simulink model "compare_serial"  (R2012b)
settings: Solver=FixedStepDiscrete  SolverMode=SingleTasking  StartTime=0.0  StopTime=5000  FixedStep=1  RelTol=1e-3
libraries: xbsIndex_r4 x1495, xps_library x1, casper_library_misc x1
(part 2 of 15)

== system compare_serial/dec_fir ==
  sync_in : Inport
  real1 : Inport  Port=2
  imag1 : Inport  Port=3
  real2 : Inport  Port=4
  imag2 : Inport  Port=5
  real3 : Inport  Port=6
  imag3 : Inport  Port=7
  real4 : Inport  Port=8
  imag4 : Inport  Port=9
  real5 : Inport  Port=10
  imag5 : Inport  Port=11
  real6 : Inport  Port=12
  imag6 : Inport  Port=13
  real7 : Inport  Port=14
  imag7 : Inport  Port=15
  real8 : Inport  Port=16
  imag8 : Inport  Port=17
  convert1 : xbsIndex_r4/Convert  gui_display_data_type=Fixed-point  arith_type="Signed  (2's comp)"  n_bits=34  bin_pt=24  float_type=Single  exp_bits=8  fraction_bits=24  quantization="Round  (unbiased: +/- Inf)"  overflow=Wrap  en=off  latency=2  dbl_ovrd=off  pipeline=off  block_type=convert
  convert2 : xbsIndex_r4/Convert  gui_display_data_type=Fixed-point  arith_type="Signed  (2's comp)"  n_bits=34  bin_pt=24  float_type=Single  exp_bits=8  fraction_bits=24  quantization="Round  (unbiased: +/- Inf)"  overflow=Wrap  en=off  latency=2  dbl_ovrd=off  pipeline=off  block_type=convert
  delay : xbsIndex_r4/Delay  rst=off  infoeditControl=Selection of Reset will increase slice count due to use of real FFs and instead of SRLs  en=off  latency=8  dbl_ovrd=off  reg_retiming=off  block_type=delay
  fir_dbl_col1 : Subsystem  AncestorBlock=casper_library_downconverter/fir_dbl_col  mask(fir_dbl_col){n_inputs=8, coeff=[3.6558e-05  8.0913e-05  0.00010847   0.0001179  0.00011054  8.9835e-05  6.0569e-05  0.00018614], add_latency=1, mult_latency=2, coeff_bit_width=16, coeff_bin_pt=15, first_stage_hdl=off, adder_imp=Behavioral}
      mask prompts: n_inputs "Inputs"; coeff "Coefficients"; add_latency "Add latency"; mult_latency "Mult Latency"; coeff_bit_width "Coefficient bit width"; coeff_bin_pt "Coefficient binary point"; first_stage_hdl "Implement first stage of adder trees on output as behavioural HDL"; adder_imp "Adder implementation"
      mask init:
      | fir_dbl_col_init(gcb, ...
      |     'n_inputs', n_inputs, ...
      |     'coeff', coeff, ...
      |     'mult_latency', mult_latency, ...
      |     'add_latency', add_latency, ...
      |     'coeff_bit_width', coeff_bit_width, ...
      |     'coeff_bin_pt', coeff_bin_pt,  ...
      |     'first_stage_hdl', first_stage_hdl, ...
      |     'adder_imp', adder_imp);
      mask Help: eval('xlWeb(''http://casper.berkeley.edu/wiki/Fir_dbl_col'')')
      mask TypeOptions adder_imp: Behavioral | Fabric | DSP48
  fir_dbl_col10 : Subsystem  AncestorBlock=casper_library_downconverter/fir_dbl_col  mask(fir_dbl_col){n_inputs=8, coeff=[-0.0039158  -0.0027465  -0.0013032  0.00020791    0.001586   0.0026617   0.0033165    0.003495], add_latency=1, mult_latency=2, coeff_bit_width=16, coeff_bin_pt=15, first_stage_hdl=off, adder_imp=Behavioral}
      mask prompts: n_inputs "Inputs"; coeff "Coefficients"; add_latency "Add latency"; mult_latency "Mult Latency"; coeff_bit_width "Coefficient bit width"; coeff_bin_pt "Coefficient binary point"; first_stage_hdl "Implement first stage of adder trees on output as behavioural HDL"; adder_imp "Adder implementation"
      mask init: same as compare_serial/dec_fir/fir_dbl_col1
      mask Help: eval('xlWeb(''http://casper.berkeley.edu/wiki/Fir_dbl_col'')')
      mask TypeOptions adder_imp: Behavioral | Fabric | DSP48
  fir_dbl_col11 : Subsystem  AncestorBlock=casper_library_downconverter/fir_dbl_col  mask(fir_dbl_col){n_inputs=8, coeff=[0.0045348   0.0026836   0.0006186  -0.0013783  -0.0030542  -0.0042152  -0.0047479  -0.0046275], add_latency=1, mult_latency=2, coeff_bit_width=16, coeff_bin_pt=15, first_stage_hdl=off, adder_imp=Behavioral}
      mask prompts: n_inputs "Inputs"; coeff "Coefficients"; add_latency "Add latency"; mult_latency "Mult Latency"; coeff_bit_width "Coefficient bit width"; coeff_bin_pt "Coefficient binary point"; first_stage_hdl "Implement first stage of adder trees on output as behavioural HDL"; adder_imp "Adder implementation"
      mask init: same as compare_serial/dec_fir/fir_dbl_col1
      mask Help: eval('xlWeb(''http://casper.berkeley.edu/wiki/Fir_dbl_col'')')
      mask TypeOptions adder_imp: Behavioral | Fabric | DSP48
  fir_dbl_col12 : Subsystem  AncestorBlock=casper_library_downconverter/fir_dbl_col  mask(fir_dbl_col){n_inputs=8, coeff=[-0.0049463  -0.0021372  0.00072915   0.0032813   0.0052161   0.0063317   0.0065461   0.0058982], add_latency=1, mult_latency=2, coeff_bit_width=16, coeff_bin_pt=15, first_stage_hdl=off, adder_imp=Behavioral}
      mask prompts: n_inputs "Inputs"; coeff "Coefficients"; add_latency "Add latency"; mult_latency "Mult Latency"; coeff_bit_width "Coefficient bit width"; coeff_bin_pt "Coefficient binary point"; first_stage_hdl "Implement first stage of adder trees on output as behavioural HDL"; adder_imp "Adder implementation"
      mask init: same as compare_serial/dec_fir/fir_dbl_col1
      mask Help: eval('xlWeb(''http://casper.berkeley.edu/wiki/Fir_dbl_col'')')
      mask TypeOptions adder_imp: Behavioral | Fabric | DSP48
  fir_dbl_col13 : Subsystem  AncestorBlock=casper_library_downconverter/fir_dbl_col  mask(fir_dbl_col){n_inputs=8, coeff=[0.0049631  0.00074424  -0.0031897  -0.0063683  -0.0084557  -0.0092805  -0.0088434  -0.0073036], add_latency=1, mult_latency=2, coeff_bit_width=16, coeff_bin_pt=15, first_stage_hdl=off, adder_imp=Behavioral}
      mask prompts: n_inputs "Inputs"; coeff "Coefficients"; add_latency "Add latency"; mult_latency "Mult Latency"; coeff_bit_width "Coefficient bit width"; coeff_bin_pt "Coefficient binary point"; first_stage_hdl "Implement first stage of adder trees on output as behavioural HDL"; adder_imp "Adder implementation"
      mask init: same as compare_serial/dec_fir/fir_dbl_col1
      mask Help: eval('xlWeb(''http://casper.berkeley.edu/wiki/Fir_dbl_col'')')
      mask TypeOptions adder_imp: Behavioral | Fabric | DSP48
  fir_dbl_col14 : Subsystem  AncestorBlock=casper_library_downconverter/fir_dbl_col  mask(fir_dbl_col){n_inputs=8, coeff=[-0.0041692   0.0024096   0.0079096    0.011788    0.013751    0.013761    0.012018   0.0089121], add_latency=1, mult_latency=2, coeff_bit_width=16, coeff_bin_pt=15, first_stage_hdl=off, adder_imp=Behavioral}
      mask prompts: n_inputs "Inputs"; coeff "Coefficients"; add_latency "Add latency"; mult_latency "Mult Latency"; coeff_bit_width "Coefficient bit width"; coeff_bin_pt "Coefficient binary point"; first_stage_hdl "Implement first stage of adder trees on output as behavioural HDL"; adder_imp "Adder implementation"
      mask init: same as compare_serial/dec_fir/fir_dbl_col1
      mask Help: eval('xlWeb(''http://casper.berkeley.edu/wiki/Fir_dbl_col'')')
      mask TypeOptions adder_imp: Behavioral | Fabric | DSP48
  fir_dbl_col15 : Subsystem  AncestorBlock=casper_library_downconverter/fir_dbl_col  mask(fir_dbl_col){n_inputs=8, coeff=[0.00081481   -0.011166   -0.019458   -0.023888   -0.024646   -0.022238   -0.017414   -0.011075], add_latency=1, mult_latency=2, coeff_bit_width=16, coeff_bin_pt=15, first_stage_hdl=off, adder_imp=Behavioral}
      mask prompts: n_inputs "Inputs"; coeff "Coefficients"; add_latency "Add latency"; mult_latency "Mult Latency"; coeff_bit_width "Coefficient bit width"; coeff_bin_pt "Coefficient binary point"; first_stage_hdl "Implement first stage of adder trees on output as behavioural HDL"; adder_imp "Adder implementation"
      mask init: same as compare_serial/dec_fir/fir_dbl_col1
      mask Help: eval('xlWeb(''http://casper.berkeley.edu/wiki/Fir_dbl_col'')')
      mask TypeOptions adder_imp: Behavioral | Fabric | DSP48
  fir_dbl_col16 : Subsystem  AncestorBlock=casper_library_downconverter/fir_dbl_col  mask(fir_dbl_col){n_inputs=8, coeff=[0.11608     0.11089     0.10094    0.087016    0.070234    0.051888    0.033353    0.015947], add_latency=1, mult_latency=2, coeff_bit_width=16, coeff_bin_pt=15, first_stage_hdl=off, adder_imp=Behavioral}
      mask prompts: n_inputs "Inputs"; coeff "Coefficients"; add_latency "Add latency"; mult_latency "Mult Latency"; coeff_bit_width "Coefficient bit width"; coeff_bin_pt "Coefficient binary point"; first_stage_hdl "Implement first stage of adder trees on output as behavioural HDL"; adder_imp "Adder implementation"
      mask init: same as compare_serial/dec_fir/fir_dbl_col1
      mask Help: eval('xlWeb(''http://casper.berkeley.edu/wiki/Fir_dbl_col'')')
      mask TypeOptions adder_imp: Behavioral | Fabric | DSP48
  fir_dbl_col2 : Subsystem  AncestorBlock=casper_library_downconverter/fir_dbl_col  mask(fir_dbl_col){n_inputs=8, coeff=[-0.0001139 -0.00017961 -0.00021408 -0.00021652 -0.00019053 -0.00014309 -8.3201e-05 -2.0412e-05], add_latency=1, mult_latency=2, coeff_bit_width=16, coeff_bin_pt=15, first_stage_hdl=off, adder_imp=Behavioral}
      mask prompts: n_inputs "Inputs"; coeff "Coefficients"; add_latency "Add latency"; mult_latency "Mult Latency"; coeff_bit_width "Coefficient bit width"; coeff_bin_pt "Coefficient binary point"; first_stage_hdl "Implement first stage of adder trees on output as behavioural HDL"; adder_imp "Adder implementation"
      mask init: same as compare_serial/dec_fir/fir_dbl_col1
      mask Help: eval('xlWeb(''http://casper.berkeley.edu/wiki/Fir_dbl_col'')')
      mask TypeOptions adder_imp: Behavioral | Fabric | DSP48
  fir_dbl_col3 : Subsystem  AncestorBlock=casper_library_downconverter/fir_dbl_col  mask(fir_dbl_col){n_inputs=8, coeff=[0.0002565  0.00034013  0.00037076  0.00035001  0.00028615  0.00019229  8.4099e-05 -2.2589e-05], add_latency=1, mult_latency=2, coeff_bit_width=16, coeff_bin_pt=15, first_stage_hdl=off, adder_imp=Behavioral}
      mask prompts: n_inputs "Inputs"; coeff "Coefficients"; add_latency "Add latency"; mult_latency "Mult Latency"; coeff_bit_width "Coefficient bit width"; coeff_bin_pt "Coefficient binary point"; first_stage_hdl "Implement first stage of adder trees on output as behavioural HDL"; adder_imp "Adder implementation"
      mask init: same as compare_serial/dec_fir/fir_dbl_col1
      mask Help: eval('xlWeb(''http://casper.berkeley.edu/wiki/Fir_dbl_col'')')
      mask TypeOptions adder_imp: Behavioral | Fabric | DSP48
  fir_dbl_col4 : Subsystem  AncestorBlock=casper_library_downconverter/fir_dbl_col  mask(fir_dbl_col){n_inputs=8, coeff=[-0.00048623 -0.00057488 -0.00058051 -0.00051035 -0.00038093 -0.00021502  -3.797e-05  0.00012591], add_latency=1, mult_latency=2, coeff_bit_width=16, coeff_bin_pt=15, first_stage_hdl=off, adder_imp=Behavioral}
      mask prompts: n_inputs "Inputs"; coeff "Coefficients"; add_latency "Add latency"; mult_latency "Mult Latency"; coeff_bit_width "Coefficient bit width"; coeff_bin_pt "Coefficient binary point"; first_stage_hdl "Implement first stage of adder trees on output as behavioural HDL"; adder_imp "Adder implementation"
      mask init: same as compare_serial/dec_fir/fir_dbl_col1
      mask Help: eval('xlWeb(''http://casper.berkeley.edu/wiki/Fir_dbl_col'')')
      mask TypeOptions adder_imp: Behavioral | Fabric | DSP48
  fir_dbl_col5 : Subsystem  AncestorBlock=casper_library_downconverter/fir_dbl_col  mask(fir_dbl_col){n_inputs=8, coeff=[0.00082138  0.00088865  0.00083479  0.00067746   0.0004464  0.00017839 -8.8198e-05 -0.00031866], add_latency=1, mult_latency=2, coeff_bit_width=16, coeff_bin_pt=15, first_stage_hdl=off, adder_imp=Behavioral}
      mask prompts: n_inputs "Inputs"; coeff "Coefficients"; add_latency "Add latency"; mult_latency "Mult Latency"; coeff_bit_width "Coefficient bit width"; coeff_bin_pt "Coefficient binary point"; first_stage_hdl "Implement first stage of adder trees on output as behavioural HDL"; adder_imp "Adder implementation"
      mask init: same as compare_serial/dec_fir/fir_dbl_col1
      mask Help: eval('xlWeb(''http://casper.berkeley.edu/wiki/Fir_dbl_col'')')
      mask TypeOptions adder_imp: Behavioral | Fabric | DSP48
  fir_dbl_col6 : Subsystem  AncestorBlock=casper_library_downconverter/fir_dbl_col  mask(fir_dbl_col){n_inputs=8, coeff=[-0.0012722  -0.0012742  -0.0011107 -0.00081658  -0.0004409 -3.9415e-05  0.00033331  0.00063107], add_latency=1, mult_latency=2, coeff_bit_width=16, coeff_bin_pt=15, first_stage_hdl=off, adder_imp=Behavioral}
      mask prompts: n_inputs "Inputs"; coeff "Coefficients"; add_latency "Add latency"; mult_latency "Mult Latency"; coeff_bit_width "Coefficient bit width"; coeff_bin_pt "Coefficient binary point"; first_stage_hdl "Implement first stage of adder trees on output as behavioural HDL"; adder_imp "Adder implementation"
      mask init: same as compare_serial/dec_fir/fir_dbl_col1
      mask Help: eval('xlWeb(''http://casper.berkeley.edu/wiki/Fir_dbl_col'')')
      mask TypeOptions adder_imp: Behavioral | Fabric | DSP48
  fir_dbl_col7 : Subsystem  AncestorBlock=casper_library_downconverter/fir_dbl_col  mask(fir_dbl_col){n_inputs=8, coeff=[0.0018361   0.0017079   0.0013679  0.00087646  0.00030942 -0.00025349  -0.0007392  -0.0010905], add_latency=1, mult_latency=2, coeff_bit_width=16, coeff_bin_pt=15, first_stage_hdl=off, adder_imp=Behavioral}
      mask prompts: n_inputs "Inputs"; coeff "Coefficients"; add_latency "Add latency"; mult_latency "Mult Latency"; coeff_bit_width "Coefficient bit width"; coeff_bin_pt "Coefficient binary point"; first_stage_hdl "Implement first stage of adder trees on output as behavioural HDL"; adder_imp "Adder implementation"
      mask init: same as compare_serial/dec_fir/fir_dbl_col1
      mask Help: eval('xlWeb(''http://casper.berkeley.edu/wiki/Fir_dbl_col'')')
      mask TypeOptions adder_imp: Behavioral | Fabric | DSP48
  fir_dbl_col8 : Subsystem  AncestorBlock=casper_library_downconverter/fir_dbl_col  mask(fir_dbl_col){n_inputs=8, coeff=[-0.0024941  -0.0021466  -0.0015457 -0.00078824   1.582e-05  0.00075832   0.0013471    0.001717], add_latency=1, mult_latency=2, coeff_bit_width=16, coeff_bin_pt=15, first_stage_hdl=off, adder_imp=Behavioral}
      mask prompts: n_inputs "Inputs"; coeff "Coefficients"; add_latency "Add latency"; mult_latency "Mult Latency"; coeff_bit_width "Coefficient bit width"; coeff_bin_pt "Coefficient binary point"; first_stage_hdl "Implement first stage of adder trees on output as behavioural HDL"; adder_imp "Adder implementation"
      mask init: same as compare_serial/dec_fir/fir_dbl_col1
      mask Help: eval('xlWeb(''http://casper.berkeley.edu/wiki/Fir_dbl_col'')')
      mask TypeOptions adder_imp: Behavioral | Fabric | DSP48
  fir_dbl_col9 : Subsystem  AncestorBlock=casper_library_downconverter/fir_dbl_col  mask(fir_dbl_col){n_inputs=8, coeff=[0.0032074   0.0025239   0.0015612  0.00046403 -0.00061536  -0.0015379  -0.0021949  -0.0025197], add_latency=1, mult_latency=2, coeff_bit_width=16, coeff_bin_pt=15, first_stage_hdl=off, adder_imp=Behavioral}
      mask prompts: n_inputs "Inputs"; coeff "Coefficients"; add_latency "Add latency"; mult_latency "Mult Latency"; coeff_bit_width "Coefficient bit width"; coeff_bin_pt "Coefficient binary point"; first_stage_hdl "Implement first stage of adder trees on output as behavioural HDL"; adder_imp "Adder implementation"
      mask init: same as compare_serial/dec_fir/fir_dbl_col1
      mask Help: eval('xlWeb(''http://casper.berkeley.edu/wiki/Fir_dbl_col'')')
      mask TypeOptions adder_imp: Behavioral | Fabric | DSP48
  imag_sum : Subsystem  AncestorBlock=casper_library_misc/adder_tree  mask(adder_tree){n_inputs=16, latency=1, adder_imp=Behavioral, first_stage_hdl=off}
      mask prompts: n_inputs "Number of Inputs"; latency "Add Latency"; adder_imp "Adder implementation"; first_stage_hdl "Use behavioural HDL for first stage of adders"
      mask help:
      | Sums all inputs using a tree of adds and delays.
      |
      | Number of inputs: The number of inputs to the block to be summed
      | Add latency: The number of clock cycles to perform one addition (affects timing)..
      | Adder implementation: choice of fabric or DSP48E core, or behavioral HDL
      | Use behavioural HDL for first stage of adders: Causes the first stage of adders to be absorbed into DSP blocks if multipliers precede them (Virtex 5). Overrides Adder implementation
      mask init:
      | adder_tree_init(gcb, ...
      |     'n_inputs', n_inputs, ...
      |     'latency', latency, ...
      |     'adder_imp', adder_imp, ...
      |     'first_stage_hdl', first_stage_hdl);
      settings: AttributesFormatString=latency 4
      mask Help: eval('xlWeb(''http://casper.berkeley.edu/wiki/Adder_tree'')')
      mask TypeOptions adder_imp: Behavioral | Fabric | DSP48
  real_sum : Subsystem  AncestorBlock=casper_library_misc/adder_tree  mask(adder_tree){n_inputs=16, latency=1, adder_imp=Behavioral, first_stage_hdl=off}
      mask prompts: n_inputs "Number of Inputs"; latency "Add Latency"; adder_imp "Adder implementation"; first_stage_hdl "Use behavioural HDL for first stage of adders"
      mask help:
      | Sums all inputs using a tree of adds and delays.
      |
      | Number of inputs: The number of inputs to the block to be summed
      | Add latency: The number of clock cycles to perform one addition (affects timing)..
      | Adder implementation: choice of fabric or DSP48E core, or behavioral HDL
      | Use behavioural HDL for first stage of adders: Causes the first stage of adders to be absorbed into DSP blocks if multipliers precede them (Virtex 5). Overrides Adder implementation
      mask init:
      | adder_tree_init(gcb, ...
      |     'n_inputs', n_inputs, ...
      |     'latency', latency, ...
      |     'adder_imp', adder_imp, ...
      |     'first_stage_hdl', first_stage_hdl);
      settings: AttributesFormatString=latency 4
      mask Help: eval('xlWeb(''http://casper.berkeley.edu/wiki/Adder_tree'')')
      mask TypeOptions adder_imp: Behavioral | Fabric | DSP48
  ri_to_c : casper_library_misc/ri_to_c
  shift1 : xbsIndex_r4/Shift  shift_dir=Left  shift_bits=0  en=off  latency=0  precision=Full  arith_type="Signed  (2's comp)"  n_bits=16  bin_pt=14  quantization=Truncate  overflow=Wrap  dbl_ovrd=off  block_type=shift
  shift2 : xbsIndex_r4/Shift  shift_dir=Left  shift_bits=0  en=off  latency=0  precision=Full  arith_type="Signed  (2's comp)"  n_bits=16  bin_pt=14  quantization=Truncate  overflow=Wrap  dbl_ovrd=off  block_type=shift
  sync_out : Outport
  dout : Outport  Port=2
  wires:
  real1/1 -> fir_dbl_col1/1(real1)
  imag1/1 -> fir_dbl_col1/2(imag1)
  real2/1 -> fir_dbl_col1/3(real2)
  imag2/1 -> fir_dbl_col1/4(imag2)
  real3/1 -> fir_dbl_col1/5(real3)
  imag3/1 -> fir_dbl_col1/6(imag3)
  real4/1 -> fir_dbl_col1/7(real4)
  imag4/1 -> fir_dbl_col1/8(imag4)
  real5/1 -> fir_dbl_col1/9(real5)
  imag5/1 -> fir_dbl_col1/10(imag5)
  real6/1 -> fir_dbl_col1/11(real6)
  imag6/1 -> fir_dbl_col1/12(imag6)
  real7/1 -> fir_dbl_col1/13(real7)
  imag7/1 -> fir_dbl_col1/14(imag7)
  real8/1 -> fir_dbl_col1/15(real8)
  imag8/1 -> fir_dbl_col1/16(imag8)
  fir_dbl_col1/33(real_sum) -> real_sum/2(din1)
  fir_dbl_col1/34(imag_sum) -> imag_sum/2(din1)
  fir_dbl_col1/1(real_out1) -> fir_dbl_col2/1(real1)
  fir_dbl_col1/2(imag_out1) -> fir_dbl_col2/2(imag1)
  fir_dbl_col1/3(real_out2) -> fir_dbl_col2/3(real2)
  fir_dbl_col1/4(imag_out2) -> fir_dbl_col2/4(imag2)
  fir_dbl_col1/5(real_out3) -> fir_dbl_col2/5(real3)
  fir_dbl_col1/6(imag_out3) -> fir_dbl_col2/6(imag3)
  fir_dbl_col1/7(real_out4) -> fir_dbl_col2/7(real4)
  fir_dbl_col1/8(imag_out4) -> fir_dbl_col2/8(imag4)
  fir_dbl_col1/9(real_out5) -> fir_dbl_col2/9(real5)
  fir_dbl_col1/10(imag_out5) -> fir_dbl_col2/10(imag5)
  fir_dbl_col1/11(real_out6) -> fir_dbl_col2/11(real6)
  fir_dbl_col1/12(imag_out6) -> fir_dbl_col2/12(imag6)
  fir_dbl_col1/13(real_out7) -> fir_dbl_col2/13(real7)
  fir_dbl_col1/14(imag_out7) -> fir_dbl_col2/14(imag7)
  fir_dbl_col1/15(real_out8) -> fir_dbl_col2/15(real8)
  fir_dbl_col1/16(imag_out8) -> fir_dbl_col2/16(imag8)
  fir_dbl_col2/33(real_sum) -> real_sum/3(din2)
  fir_dbl_col2/34(imag_sum) -> imag_sum/3(din2)
  fir_dbl_col2/1(real_out1) -> fir_dbl_col3/1(real1)
  fir_dbl_col2/2(imag_out1) -> fir_dbl_col3/2(imag1)
  fir_dbl_col2/3(real_out2) -> fir_dbl_col3/3(real2)
  fir_dbl_col2/4(imag_out2) -> fir_dbl_col3/4(imag2)
  fir_dbl_col2/5(real_out3) -> fir_dbl_col3/5(real3)
  fir_dbl_col2/6(imag_out3) -> fir_dbl_col3/6(imag3)
  fir_dbl_col2/7(real_out4) -> fir_dbl_col3/7(real4)
  fir_dbl_col2/8(imag_out4) -> fir_dbl_col3/8(imag4)
  fir_dbl_col2/9(real_out5) -> fir_dbl_col3/9(real5)
  fir_dbl_col2/10(imag_out5) -> fir_dbl_col3/10(imag5)
  fir_dbl_col2/11(real_out6) -> fir_dbl_col3/11(real6)
  fir_dbl_col2/12(imag_out6) -> fir_dbl_col3/12(imag6)
  fir_dbl_col2/13(real_out7) -> fir_dbl_col3/13(real7)
  fir_dbl_col2/14(imag_out7) -> fir_dbl_col3/14(imag7)
  fir_dbl_col2/15(real_out8) -> fir_dbl_col3/15(real8)
  fir_dbl_col2/16(imag_out8) -> fir_dbl_col3/16(imag8)
  fir_dbl_col3/33(real_sum) -> real_sum/4(din3)
  fir_dbl_col3/34(imag_sum) -> imag_sum/4(din3)
  fir_dbl_col3/1(real_out1) -> fir_dbl_col4/1(real1)
  fir_dbl_col3/2(imag_out1) -> fir_dbl_col4/2(imag1)
  fir_dbl_col3/3(real_out2) -> fir_dbl_col4/3(real2)
  fir_dbl_col3/4(imag_out2) -> fir_dbl_col4/4(imag2)
  fir_dbl_col3/5(real_out3) -> fir_dbl_col4/5(real3)
  fir_dbl_col3/6(imag_out3) -> fir_dbl_col4/6(imag3)
  fir_dbl_col3/7(real_out4) -> fir_dbl_col4/7(real4)
  fir_dbl_col3/8(imag_out4) -> fir_dbl_col4/8(imag4)
  fir_dbl_col3/9(real_out5) -> fir_dbl_col4/9(real5)
  fir_dbl_col3/10(imag_out5) -> fir_dbl_col4/10(imag5)
  fir_dbl_col3/11(real_out6) -> fir_dbl_col4/11(real6)
  fir_dbl_col3/12(imag_out6) -> fir_dbl_col4/12(imag6)
  fir_dbl_col3/13(real_out7) -> fir_dbl_col4/13(real7)
  fir_dbl_col3/14(imag_out7) -> fir_dbl_col4/14(imag7)
  fir_dbl_col3/15(real_out8) -> fir_dbl_col4/15(real8)
  fir_dbl_col3/16(imag_out8) -> fir_dbl_col4/16(imag8)
  fir_dbl_col4/33(real_sum) -> real_sum/5(din4)
  fir_dbl_col4/34(imag_sum) -> imag_sum/5(din4)
  fir_dbl_col4/1(real_out1) -> fir_dbl_col5/1(real1)
  fir_dbl_col4/2(imag_out1) -> fir_dbl_col5/2(imag1)
  fir_dbl_col4/3(real_out2) -> fir_dbl_col5/3(real2)
  fir_dbl_col4/4(imag_out2) -> fir_dbl_col5/4(imag2)
  fir_dbl_col4/5(real_out3) -> fir_dbl_col5/5(real3)
  fir_dbl_col4/6(imag_out3) -> fir_dbl_col5/6(imag3)
  fir_dbl_col4/7(real_out4) -> fir_dbl_col5/7(real4)
  fir_dbl_col4/8(imag_out4) -> fir_dbl_col5/8(imag4)
  fir_dbl_col4/9(real_out5) -> fir_dbl_col5/9(real5)
  fir_dbl_col4/10(imag_out5) -> fir_dbl_col5/10(imag5)
  fir_dbl_col4/11(real_out6) -> fir_dbl_col5/11(real6)
  fir_dbl_col4/12(imag_out6) -> fir_dbl_col5/12(imag6)
  fir_dbl_col4/13(real_out7) -> fir_dbl_col5/13(real7)
  fir_dbl_col4/14(imag_out7) -> fir_dbl_col5/14(imag7)
  fir_dbl_col4/15(real_out8) -> fir_dbl_col5/15(real8)
  fir_dbl_col4/16(imag_out8) -> fir_dbl_col5/16(imag8)
  fir_dbl_col5/33(real_sum) -> real_sum/6(din5)
  fir_dbl_col5/34(imag_sum) -> imag_sum/6(din5)
  fir_dbl_col5/1(real_out1) -> fir_dbl_col6/1(real1)
  fir_dbl_col5/2(imag_out1) -> fir_dbl_col6/2(imag1)
  fir_dbl_col5/3(real_out2) -> fir_dbl_col6/3(real2)
  fir_dbl_col5/4(imag_out2) -> fir_dbl_col6/4(imag2)
  fir_dbl_col5/5(real_out3) -> fir_dbl_col6/5(real3)
  fir_dbl_col5/6(imag_out3) -> fir_dbl_col6/6(imag3)
  fir_dbl_col5/7(real_out4) -> fir_dbl_col6/7(real4)
  fir_dbl_col5/8(imag_out4) -> fir_dbl_col6/8(imag4)
  fir_dbl_col5/9(real_out5) -> fir_dbl_col6/9(real5)
  fir_dbl_col5/10(imag_out5) -> fir_dbl_col6/10(imag5)
  fir_dbl_col5/11(real_out6) -> fir_dbl_col6/11(real6)
  fir_dbl_col5/12(imag_out6) -> fir_dbl_col6/12(imag6)
  fir_dbl_col5/13(real_out7) -> fir_dbl_col6/13(real7)
  fir_dbl_col5/14(imag_out7) -> fir_dbl_col6/14(imag7)
  fir_dbl_col5/15(real_out8) -> fir_dbl_col6/15(real8)
  fir_dbl_col5/16(imag_out8) -> fir_dbl_col6/16(imag8)
  fir_dbl_col6/33(real_sum) -> real_sum/7(din6)
  fir_dbl_col6/34(imag_sum) -> imag_sum/7(din6)
  fir_dbl_col6/1(real_out1) -> fir_dbl_col7/1(real1)
  fir_dbl_col6/2(imag_out1) -> fir_dbl_col7/2(imag1)
  fir_dbl_col6/3(real_out2) -> fir_dbl_col7/3(real2)
  fir_dbl_col6/4(imag_out2) -> fir_dbl_col7/4(imag2)
  fir_dbl_col6/5(real_out3) -> fir_dbl_col7/5(real3)
  fir_dbl_col6/6(imag_out3) -> fir_dbl_col7/6(imag3)
  fir_dbl_col6/7(real_out4) -> fir_dbl_col7/7(real4)
  fir_dbl_col6/8(imag_out4) -> fir_dbl_col7/8(imag4)
  fir_dbl_col6/9(real_out5) -> fir_dbl_col7/9(real5)
  fir_dbl_col6/10(imag_out5) -> fir_dbl_col7/10(imag5)
  fir_dbl_col6/11(real_out6) -> fir_dbl_col7/11(real6)
  fir_dbl_col6/12(imag_out6) -> fir_dbl_col7/12(imag6)
  fir_dbl_col6/13(real_out7) -> fir_dbl_col7/13(real7)
  fir_dbl_col6/14(imag_out7) -> fir_dbl_col7/14(imag7)
  fir_dbl_col6/15(real_out8) -> fir_dbl_col7/15(real8)
  fir_dbl_col6/16(imag_out8) -> fir_dbl_col7/16(imag8)
  fir_dbl_col7/33(real_sum) -> real_sum/8(din7)
  fir_dbl_col7/34(imag_sum) -> imag_sum/8(din7)
  fir_dbl_col7/1(real_out1) -> fir_dbl_col8/1(real1)
  fir_dbl_col7/2(imag_out1) -> fir_dbl_col8/2(imag1)
  fir_dbl_col7/3(real_out2) -> fir_dbl_col8/3(real2)
  fir_dbl_col7/4(imag_out2) -> fir_dbl_col8/4(imag2)
  fir_dbl_col7/5(real_out3) -> fir_dbl_col8/5(real3)
  fir_dbl_col7/6(imag_out3) -> fir_dbl_col8/6(imag3)
  fir_dbl_col7/7(real_out4) -> fir_dbl_col8/7(real4)
  fir_dbl_col7/8(imag_out4) -> fir_dbl_col8/8(imag4)
  fir_dbl_col7/9(real_out5) -> fir_dbl_col8/9(real5)
  fir_dbl_col7/10(imag_out5) -> fir_dbl_col8/10(imag5)
  fir_dbl_col7/11(real_out6) -> fir_dbl_col8/11(real6)
  fir_dbl_col7/12(imag_out6) -> fir_dbl_col8/12(imag6)
  fir_dbl_col7/13(real_out7) -> fir_dbl_col8/13(real7)
  fir_dbl_col7/14(imag_out7) -> fir_dbl_col8/14(imag7)
  fir_dbl_col7/15(real_out8) -> fir_dbl_col8/15(real8)
  fir_dbl_col7/16(imag_out8) -> fir_dbl_col8/16(imag8)
  fir_dbl_col8/33(real_sum) -> real_sum/9(din8)
  fir_dbl_col8/34(imag_sum) -> imag_sum/9(din8)
  fir_dbl_col8/1(real_out1) -> fir_dbl_col9/1(real1)
  fir_dbl_col8/2(imag_out1) -> fir_dbl_col9/2(imag1)
  fir_dbl_col8/3(real_out2) -> fir_dbl_col9/3(real2)
  fir_dbl_col8/4(imag_out2) -> fir_dbl_col9/4(imag2)
  fir_dbl_col8/5(real_out3) -> fir_dbl_col9/5(real3)
  fir_dbl_col8/6(imag_out3) -> fir_dbl_col9/6(imag3)
  fir_dbl_col8/7(real_out4) -> fir_dbl_col9/7(real4)
  fir_dbl_col8/8(imag_out4) -> fir_dbl_col9/8(imag4)
  fir_dbl_col8/9(real_out5) -> fir_dbl_col9/9(real5)
  fir_dbl_col8/10(imag_out5) -> fir_dbl_col9/10(imag5)
  fir_dbl_col8/11(real_out6) -> fir_dbl_col9/11(real6)
  fir_dbl_col8/12(imag_out6) -> fir_dbl_col9/12(imag6)
  fir_dbl_col8/13(real_out7) -> fir_dbl_col9/13(real7)
  fir_dbl_col8/14(imag_out7) -> fir_dbl_col9/14(imag7)
  fir_dbl_col8/15(real_out8) -> fir_dbl_col9/15(real8)
  fir_dbl_col8/16(imag_out8) -> fir_dbl_col9/16(imag8)
  fir_dbl_col9/33(real_sum) -> real_sum/10(din9)
  fir_dbl_col9/34(imag_sum) -> imag_sum/10(din9)
  fir_dbl_col9/1(real_out1) -> fir_dbl_col10/1(real1)
  fir_dbl_col9/2(imag_out1) -> fir_dbl_col10/2(imag1)
  fir_dbl_col9/3(real_out2) -> fir_dbl_col10/3(real2)
  fir_dbl_col9/4(imag_out2) -> fir_dbl_col10/4(imag2)
  fir_dbl_col9/5(real_out3) -> fir_dbl_col10/5(real3)
  fir_dbl_col9/6(imag_out3) -> fir_dbl_col10/6(imag3)
  fir_dbl_col9/7(real_out4) -> fir_dbl_col10/7(real4)
  fir_dbl_col9/8(imag_out4) -> fir_dbl_col10/8(imag4)
  fir_dbl_col9/9(real_out5) -> fir_dbl_col10/9(real5)
  fir_dbl_col9/10(imag_out5) -> fir_dbl_col10/10(imag5)
  fir_dbl_col9/11(real_out6) -> fir_dbl_col10/11(real6)
  fir_dbl_col9/12(imag_out6) -> fir_dbl_col10/12(imag6)
  fir_dbl_col9/13(real_out7) -> fir_dbl_col10/13(real7)
  fir_dbl_col9/14(imag_out7) -> fir_dbl_col10/14(imag7)
  fir_dbl_col9/15(real_out8) -> fir_dbl_col10/15(real8)
  fir_dbl_col9/16(imag_out8) -> fir_dbl_col10/16(imag8)
  fir_dbl_col10/33(real_sum) -> real_sum/11(din10)
  fir_dbl_col10/34(imag_sum) -> imag_sum/11(din10)
  fir_dbl_col10/1(real_out1) -> fir_dbl_col11/1(real1)
  fir_dbl_col10/2(imag_out1) -> fir_dbl_col11/2(imag1)
  fir_dbl_col10/3(real_out2) -> fir_dbl_col11/3(real2)
  fir_dbl_col10/4(imag_out2) -> fir_dbl_col11/4(imag2)
  fir_dbl_col10/5(real_out3) -> fir_dbl_col11/5(real3)
  fir_dbl_col10/6(imag_out3) -> fir_dbl_col11/6(imag3)
  fir_dbl_col10/7(real_out4) -> fir_dbl_col11/7(real4)
  fir_dbl_col10/8(imag_out4) -> fir_dbl_col11/8(imag4)
  fir_dbl_col10/9(real_out5) -> fir_dbl_col11/9(real5)
  fir_dbl_col10/10(imag_out5) -> fir_dbl_col11/10(imag5)
  fir_dbl_col10/11(real_out6) -> fir_dbl_col11/11(real6)
  fir_dbl_col10/12(imag_out6) -> fir_dbl_col11/12(imag6)
  fir_dbl_col10/13(real_out7) -> fir_dbl_col11/13(real7)
  fir_dbl_col10/14(imag_out7) -> fir_dbl_col11/14(imag7)
  fir_dbl_col10/15(real_out8) -> fir_dbl_col11/15(real8)
  fir_dbl_col10/16(imag_out8) -> fir_dbl_col11/16(imag8)
  fir_dbl_col11/33(real_sum) -> real_sum/12(din11)
  fir_dbl_col11/34(imag_sum) -> imag_sum/12(din11)
  fir_dbl_col11/1(real_out1) -> fir_dbl_col12/1(real1)
  fir_dbl_col11/2(imag_out1) -> fir_dbl_col12/2(imag1)
  fir_dbl_col11/3(real_out2) -> fir_dbl_col12/3(real2)
  fir_dbl_col11/4(imag_out2) -> fir_dbl_col12/4(imag2)
  fir_dbl_col11/5(real_out3) -> fir_dbl_col12/5(real3)
  fir_dbl_col11/6(imag_out3) -> fir_dbl_col12/6(imag3)
  fir_dbl_col11/7(real_out4) -> fir_dbl_col12/7(real4)
  fir_dbl_col11/8(imag_out4) -> fir_dbl_col12/8(imag4)
  fir_dbl_col11/9(real_out5) -> fir_dbl_col12/9(real5)
  fir_dbl_col11/10(imag_out5) -> fir_dbl_col12/10(imag5)
  fir_dbl_col11/11(real_out6) -> fir_dbl_col12/11(real6)
  fir_dbl_col11/12(imag_out6) -> fir_dbl_col12/12(imag6)
  fir_dbl_col11/13(real_out7) -> fir_dbl_col12/13(real7)
  fir_dbl_col11/14(imag_out7) -> fir_dbl_col12/14(imag7)
  fir_dbl_col11/15(real_out8) -> fir_dbl_col12/15(real8)
  fir_dbl_col11/16(imag_out8) -> fir_dbl_col12/16(imag8)
  fir_dbl_col12/33(real_sum) -> real_sum/13(din12)
  fir_dbl_col12/34(imag_sum) -> imag_sum/13(din12)
  fir_dbl_col12/1(real_out1) -> fir_dbl_col13/1(real1)
  fir_dbl_col12/2(imag_out1) -> fir_dbl_col13/2(imag1)
  fir_dbl_col12/3(real_out2) -> fir_dbl_col13/3(real2)
  fir_dbl_col12/4(imag_out2) -> fir_dbl_col13/4(imag2)
  fir_dbl_col12/5(real_out3) -> fir_dbl_col13/5(real3)
  fir_dbl_col12/6(imag_out3) -> fir_dbl_col13/6(imag3)
  fir_dbl_col12/7(real_out4) -> fir_dbl_col13/7(real4)
  fir_dbl_col12/8(imag_out4) -> fir_dbl_col13/8(imag4)
  fir_dbl_col12/9(real_out5) -> fir_dbl_col13/9(real5)
  fir_dbl_col12/10(imag_out5) -> fir_dbl_col13/10(imag5)
  fir_dbl_col12/11(real_out6) -> fir_dbl_col13/11(real6)
  fir_dbl_col12/12(imag_out6) -> fir_dbl_col13/12(imag6)
  fir_dbl_col12/13(real_out7) -> fir_dbl_col13/13(real7)
  fir_dbl_col12/14(imag_out7) -> fir_dbl_col13/14(imag7)
  fir_dbl_col12/15(real_out8) -> fir_dbl_col13/15(real8)
  fir_dbl_col12/16(imag_out8) -> fir_dbl_col13/16(imag8)
  fir_dbl_col13/33(real_sum) -> real_sum/14(din13)
  fir_dbl_col13/34(imag_sum) -> imag_sum/14(din13)
  fir_dbl_col13/1(real_out1) -> fir_dbl_col14/1(real1)
  fir_dbl_col13/2(imag_out1) -> fir_dbl_col14/2(imag1)
  fir_dbl_col13/3(real_out2) -> fir_dbl_col14/3(real2)
  fir_dbl_col13/4(imag_out2) -> fir_dbl_col14/4(imag2)
  fir_dbl_col13/5(real_out3) -> fir_dbl_col14/5(real3)
  fir_dbl_col13/6(imag_out3) -> fir_dbl_col14/6(imag3)
  fir_dbl_col13/7(real_out4) -> fir_dbl_col14/7(real4)
  fir_dbl_col13/8(imag_out4) -> fir_dbl_col14/8(imag4)
  fir_dbl_col13/9(real_out5) -> fir_dbl_col14/9(real5)
  fir_dbl_col13/10(imag_out5) -> fir_dbl_col14/10(imag5)
  fir_dbl_col13/11(real_out6) -> fir_dbl_col14/11(real6)
  fir_dbl_col13/12(imag_out6) -> fir_dbl_col14/12(imag6)
  fir_dbl_col13/13(real_out7) -> fir_dbl_col14/13(real7)
  fir_dbl_col13/14(imag_out7) -> fir_dbl_col14/14(imag7)
  fir_dbl_col13/15(real_out8) -> fir_dbl_col14/15(real8)
  fir_dbl_col13/16(imag_out8) -> fir_dbl_col14/16(imag8)
  fir_dbl_col14/33(real_sum) -> real_sum/15(din14)
  fir_dbl_col14/34(imag_sum) -> imag_sum/15(din14)
  fir_dbl_col14/1(real_out1) -> fir_dbl_col15/1(real1)
  fir_dbl_col14/2(imag_out1) -> fir_dbl_col15/2(imag1)
  fir_dbl_col14/3(real_out2) -> fir_dbl_col15/3(real2)
  fir_dbl_col14/4(imag_out2) -> fir_dbl_col15/4(imag2)
  fir_dbl_col14/5(real_out3) -> fir_dbl_col15/5(real3)
  fir_dbl_col14/6(imag_out3) -> fir_dbl_col15/6(imag3)
  fir_dbl_col14/7(real_out4) -> fir_dbl_col15/7(real4)
  fir_dbl_col14/8(imag_out4) -> fir_dbl_col15/8(imag4)
  fir_dbl_col14/9(real_out5) -> fir_dbl_col15/9(real5)
  fir_dbl_col14/10(imag_out5) -> fir_dbl_col15/10(imag5)
  fir_dbl_col14/11(real_out6) -> fir_dbl_col15/11(real6)
  fir_dbl_col14/12(imag_out6) -> fir_dbl_col15/12(imag6)
  fir_dbl_col14/13(real_out7) -> fir_dbl_col15/13(real7)
  fir_dbl_col14/14(imag_out7) -> fir_dbl_col15/14(imag7)
  fir_dbl_col14/15(real_out8) -> fir_dbl_col15/15(real8)
  fir_dbl_col14/16(imag_out8) -> fir_dbl_col15/16(imag8)
  fir_dbl_col15/33(real_sum) -> real_sum/16(din15)
  fir_dbl_col15/34(imag_sum) -> imag_sum/16(din15)
  fir_dbl_col15/1(real_out1) -> fir_dbl_col16/1(real1)
  fir_dbl_col15/2(imag_out1) -> fir_dbl_col16/2(imag1)
  fir_dbl_col15/3(real_out2) -> fir_dbl_col16/3(real2)
  fir_dbl_col15/4(imag_out2) -> fir_dbl_col16/4(imag2)
  fir_dbl_col15/5(real_out3) -> fir_dbl_col16/5(real3)
  fir_dbl_col15/6(imag_out3) -> fir_dbl_col16/6(imag3)
  fir_dbl_col15/7(real_out4) -> fir_dbl_col16/7(real4)
  fir_dbl_col15/8(imag_out4) -> fir_dbl_col16/8(imag4)
  fir_dbl_col15/9(real_out5) -> fir_dbl_col16/9(real5)
  fir_dbl_col15/10(imag_out5) -> fir_dbl_col16/10(imag5)
  fir_dbl_col15/11(real_out6) -> fir_dbl_col16/11(real6)
  fir_dbl_col15/12(imag_out6) -> fir_dbl_col16/12(imag6)
  fir_dbl_col15/13(real_out7) -> fir_dbl_col16/13(real7)
  fir_dbl_col15/14(imag_out7) -> fir_dbl_col16/14(imag7)
  fir_dbl_col15/15(real_out8) -> fir_dbl_col16/15(real8)
  fir_dbl_col15/16(imag_out8) -> fir_dbl_col16/16(imag8)
  fir_dbl_col16/33(real_sum) -> real_sum/17(din16)
  fir_dbl_col16/34(imag_sum) -> imag_sum/17(din16)
  real_sum/2(dout) -> shift1/1
  imag_sum/2(dout) -> shift2/1
  shift1/1 -> convert1/1
  shift2/1 -> convert2/1
  convert1/1 -> ri_to_c/1
  convert2/1 -> ri_to_c/2
  ri_to_c/1 -> dout/1
  sync_in/1 -> delay/1
  delay/1 -> real_sum/1(sync), imag_sum/1(sync)
  real_sum/1(sync_out) -> sync_out/1
  fir_dbl_col2/17(real_back_out1) -> fir_dbl_col1/17(real_back1)
  fir_dbl_col2/18(imag_back_out1) -> fir_dbl_col1/18(imag_back1)
  fir_dbl_col2/19(real_back_out2) -> fir_dbl_col1/19(real_back2)
  fir_dbl_col2/20(imag_back_out2) -> fir_dbl_col1/20(imag_back2)
  fir_dbl_col2/21(real_back_out3) -> fir_dbl_col1/21(real_back3)
  fir_dbl_col2/22(imag_back_out3) -> fir_dbl_col1/22(imag_back3)
  fir_dbl_col2/23(real_back_out4) -> fir_dbl_col1/23(real_back4)
  fir_dbl_col2/24(imag_back_out4) -> fir_dbl_col1/24(imag_back4)
  fir_dbl_col2/25(real_back_out5) -> fir_dbl_col1/25(real_back5)
  fir_dbl_col2/26(imag_back_out5) -> fir_dbl_col1/26(imag_back5)
  fir_dbl_col2/27(real_back_out6) -> fir_dbl_col1/27(real_back6)
  fir_dbl_col2/28(imag_back_out6) -> fir_dbl_col1/28(imag_back6)
  fir_dbl_col2/29(real_back_out7) -> fir_dbl_col1/29(real_back7)
  fir_dbl_col2/30(imag_back_out7) -> fir_dbl_col1/30(imag_back7)
  fir_dbl_col2/31(real_back_out8) -> fir_dbl_col1/31(real_back8)
  fir_dbl_col2/32(imag_back_out8) -> fir_dbl_col1/32(imag_back8)
  fir_dbl_col3/17(real_back_out1) -> fir_dbl_col2/17(real_back1)
  fir_dbl_col3/18(imag_back_out1) -> fir_dbl_col2/18(imag_back1)
  fir_dbl_col3/19(real_back_out2) -> fir_dbl_col2/19(real_back2)
  fir_dbl_col3/20(imag_back_out2) -> fir_dbl_col2/20(imag_back2)
  fir_dbl_col3/21(real_back_out3) -> fir_dbl_col2/21(real_back3)
  fir_dbl_col3/22(imag_back_out3) -> fir_dbl_col2/22(imag_back3)
  fir_dbl_col3/23(real_back_out4) -> fir_dbl_col2/23(real_back4)
  fir_dbl_col3/24(imag_back_out4) -> fir_dbl_col2/24(imag_back4)
  fir_dbl_col3/25(real_back_out5) -> fir_dbl_col2/25(real_back5)
  fir_dbl_col3/26(imag_back_out5) -> fir_dbl_col2/26(imag_back5)
  fir_dbl_col3/27(real_back_out6) -> fir_dbl_col2/27(real_back6)
  fir_dbl_col3/28(imag_back_out6) -> fir_dbl_col2/28(imag_back6)
  fir_dbl_col3/29(real_back_out7) -> fir_dbl_col2/29(real_back7)
  fir_dbl_col3/30(imag_back_out7) -> fir_dbl_col2/30(imag_back7)
  fir_dbl_col3/31(real_back_out8) -> fir_dbl_col2/31(real_back8)
  fir_dbl_col3/32(imag_back_out8) -> fir_dbl_col2/32(imag_back8)
  fir_dbl_col4/17(real_back_out1) -> fir_dbl_col3/17(real_back1)
  fir_dbl_col4/18(imag_back_out1) -> fir_dbl_col3/18(imag_back1)
  fir_dbl_col4/19(real_back_out2) -> fir_dbl_col3/19(real_back2)
  fir_dbl_col4/20(imag_back_out2) -> fir_dbl_col3/20(imag_back2)
  fir_dbl_col4/21(real_back_out3) -> fir_dbl_col3/21(real_back3)
  fir_dbl_col4/22(imag_back_out3) -> fir_dbl_col3/22(imag_back3)
  fir_dbl_col4/23(real_back_out4) -> fir_dbl_col3/23(real_back4)
  fir_dbl_col4/24(imag_back_out4) -> fir_dbl_col3/24(imag_back4)
  fir_dbl_col4/25(real_back_out5) -> fir_dbl_col3/25(real_back5)
  fir_dbl_col4/26(imag_back_out5) -> fir_dbl_col3/26(imag_back5)
  fir_dbl_col4/27(real_back_out6) -> fir_dbl_col3/27(real_back6)
  fir_dbl_col4/28(imag_back_out6) -> fir_dbl_col3/28(imag_back6)
  fir_dbl_col4/29(real_back_out7) -> fir_dbl_col3/29(real_back7)
  fir_dbl_col4/30(imag_back_out7) -> fir_dbl_col3/30(imag_back7)
  fir_dbl_col4/31(real_back_out8) -> fir_dbl_col3/31(real_back8)
  fir_dbl_col4/32(imag_back_out8) -> fir_dbl_col3/32(imag_back8)
  fir_dbl_col5/17(real_back_out1) -> fir_dbl_col4/17(real_back1)
  fir_dbl_col5/18(imag_back_out1) -> fir_dbl_col4/18(imag_back1)
  fir_dbl_col5/19(real_back_out2) -> fir_dbl_col4/19(real_back2)
  fir_dbl_col5/20(imag_back_out2) -> fir_dbl_col4/20(imag_back2)
  fir_dbl_col5/21(real_back_out3) -> fir_dbl_col4/21(real_back3)
  fir_dbl_col5/22(imag_back_out3) -> fir_dbl_col4/22(imag_back3)
  fir_dbl_col5/23(real_back_out4) -> fir_dbl_col4/23(real_back4)
  fir_dbl_col5/24(imag_back_out4) -> fir_dbl_col4/24(imag_back4)
  fir_dbl_col5/25(real_back_out5) -> fir_dbl_col4/25(real_back5)
  fir_dbl_col5/26(imag_back_out5) -> fir_dbl_col4/26(imag_back5)
  fir_dbl_col5/27(real_back_out6) -> fir_dbl_col4/27(real_back6)
  fir_dbl_col5/28(imag_back_out6) -> fir_dbl_col4/28(imag_back6)
  fir_dbl_col5/29(real_back_out7) -> fir_dbl_col4/29(real_back7)
  fir_dbl_col5/30(imag_back_out7) -> fir_dbl_col4/30(imag_back7)
  fir_dbl_col5/31(real_back_out8) -> fir_dbl_col4/31(real_back8)
  fir_dbl_col5/32(imag_back_out8) -> fir_dbl_col4/32(imag_back8)
  fir_dbl_col6/17(real_back_out1) -> fir_dbl_col5/17(real_back1)
  fir_dbl_col6/18(imag_back_out1) -> fir_dbl_col5/18(imag_back1)
  fir_dbl_col6/19(real_back_out2) -> fir_dbl_col5/19(real_back2)
  fir_dbl_col6/20(imag_back_out2) -> fir_dbl_col5/20(imag_back2)
  fir_dbl_col6/21(real_back_out3) -> fir_dbl_col5/21(real_back3)
  fir_dbl_col6/22(imag_back_out3) -> fir_dbl_col5/22(imag_back3)
  fir_dbl_col6/23(real_back_out4) -> fir_dbl_col5/23(real_back4)
  fir_dbl_col6/24(imag_back_out4) -> fir_dbl_col5/24(imag_back4)
  fir_dbl_col6/25(real_back_out5) -> fir_dbl_col5/25(real_back5)
  fir_dbl_col6/26(imag_back_out5) -> fir_dbl_col5/26(imag_back5)
  fir_dbl_col6/27(real_back_out6) -> fir_dbl_col5/27(real_back6)
  fir_dbl_col6/28(imag_back_out6) -> fir_dbl_col5/28(imag_back6)
  fir_dbl_col6/29(real_back_out7) -> fir_dbl_col5/29(real_back7)
  fir_dbl_col6/30(imag_back_out7) -> fir_dbl_col5/30(imag_back7)
  fir_dbl_col6/31(real_back_out8) -> fir_dbl_col5/31(real_back8)
  fir_dbl_col6/32(imag_back_out8) -> fir_dbl_col5/32(imag_back8)
  fir_dbl_col7/17(real_back_out1) -> fir_dbl_col6/17(real_back1)
  fir_dbl_col7/18(imag_back_out1) -> fir_dbl_col6/18(imag_back1)
  fir_dbl_col7/19(real_back_out2) -> fir_dbl_col6/19(real_back2)
  fir_dbl_col7/20(imag_back_out2) -> fir_dbl_col6/20(imag_back2)
  fir_dbl_col7/21(real_back_out3) -> fir_dbl_col6/21(real_back3)
  fir_dbl_col7/22(imag_back_out3) -> fir_dbl_col6/22(imag_back3)
  fir_dbl_col7/23(real_back_out4) -> fir_dbl_col6/23(real_back4)
  fir_dbl_col7/24(imag_back_out4) -> fir_dbl_col6/24(imag_back4)
  fir_dbl_col7/25(real_back_out5) -> fir_dbl_col6/25(real_back5)
  fir_dbl_col7/26(imag_back_out5) -> fir_dbl_col6/26(imag_back5)
  fir_dbl_col7/27(real_back_out6) -> fir_dbl_col6/27(real_back6)
  fir_dbl_col7/28(imag_back_out6) -> fir_dbl_col6/28(imag_back6)
  fir_dbl_col7/29(real_back_out7) -> fir_dbl_col6/29(real_back7)
  fir_dbl_col7/30(imag_back_out7) -> fir_dbl_col6/30(imag_back7)
  fir_dbl_col7/31(real_back_out8) -> fir_dbl_col6/31(real_back8)
  fir_dbl_col7/32(imag_back_out8) -> fir_dbl_col6/32(imag_back8)
  fir_dbl_col8/17(real_back_out1) -> fir_dbl_col7/17(real_back1)
  fir_dbl_col8/18(imag_back_out1) -> fir_dbl_col7/18(imag_back1)
  fir_dbl_col8/19(real_back_out2) -> fir_dbl_col7/19(real_back2)
  fir_dbl_col8/20(imag_back_out2) -> fir_dbl_col7/20(imag_back2)
  fir_dbl_col8/21(real_back_out3) -> fir_dbl_col7/21(real_back3)
  fir_dbl_col8/22(imag_back_out3) -> fir_dbl_col7/22(imag_back3)
  fir_dbl_col8/23(real_back_out4) -> fir_dbl_col7/23(real_back4)
  fir_dbl_col8/24(imag_back_out4) -> fir_dbl_col7/24(imag_back4)
  fir_dbl_col8/25(real_back_out5) -> fir_dbl_col7/25(real_back5)
  fir_dbl_col8/26(imag_back_out5) -> fir_dbl_col7/26(imag_back5)
  fir_dbl_col8/27(real_back_out6) -> fir_dbl_col7/27(real_back6)
  fir_dbl_col8/28(imag_back_out6) -> fir_dbl_col7/28(imag_back6)
  fir_dbl_col8/29(real_back_out7) -> fir_dbl_col7/29(real_back7)
  fir_dbl_col8/30(imag_back_out7) -> fir_dbl_col7/30(imag_back7)
  fir_dbl_col8/31(real_back_out8) -> fir_dbl_col7/31(real_back8)
  fir_dbl_col8/32(imag_back_out8) -> fir_dbl_col7/32(imag_back8)
  fir_dbl_col9/17(real_back_out1) -> fir_dbl_col8/17(real_back1)
  fir_dbl_col9/18(imag_back_out1) -> fir_dbl_col8/18(imag_back1)
  fir_dbl_col9/19(real_back_out2) -> fir_dbl_col8/19(real_back2)
  fir_dbl_col9/20(imag_back_out2) -> fir_dbl_col8/20(imag_back2)
  fir_dbl_col9/21(real_back_out3) -> fir_dbl_col8/21(real_back3)
  fir_dbl_col9/22(imag_back_out3) -> fir_dbl_col8/22(imag_back3)
  fir_dbl_col9/23(real_back_out4) -> fir_dbl_col8/23(real_back4)
  fir_dbl_col9/24(imag_back_out4) -> fir_dbl_col8/24(imag_back4)
  fir_dbl_col9/25(real_back_out5) -> fir_dbl_col8/25(real_back5)
  fir_dbl_col9/26(imag_back_out5) -> fir_dbl_col8/26(imag_back5)
  fir_dbl_col9/27(real_back_out6) -> fir_dbl_col8/27(real_back6)
  fir_dbl_col9/28(imag_back_out6) -> fir_dbl_col8/28(imag_back6)
  fir_dbl_col9/29(real_back_out7) -> fir_dbl_col8/29(real_back7)
  fir_dbl_col9/30(imag_back_out7) -> fir_dbl_col8/30(imag_back7)
  fir_dbl_col9/31(real_back_out8) -> fir_dbl_col8/31(real_back8)
  fir_dbl_col9/32(imag_back_out8) -> fir_dbl_col8/32(imag_back8)
  fir_dbl_col10/17(real_back_out1) -> fir_dbl_col9/17(real_back1)
  fir_dbl_col10/18(imag_back_out1) -> fir_dbl_col9/18(imag_back1)
  fir_dbl_col10/19(real_back_out2) -> fir_dbl_col9/19(real_back2)
  fir_dbl_col10/20(imag_back_out2) -> fir_dbl_col9/20(imag_back2)
  fir_dbl_col10/21(real_back_out3) -> fir_dbl_col9/21(real_back3)
  fir_dbl_col10/22(imag_back_out3) -> fir_dbl_col9/22(imag_back3)
  fir_dbl_col10/23(real_back_out4) -> fir_dbl_col9/23(real_back4)
  fir_dbl_col10/24(imag_back_out4) -> fir_dbl_col9/24(imag_back4)
  fir_dbl_col10/25(real_back_out5) -> fir_dbl_col9/25(real_back5)
  fir_dbl_col10/26(imag_back_out5) -> fir_dbl_col9/26(imag_back5)
  fir_dbl_col10/27(real_back_out6) -> fir_dbl_col9/27(real_back6)
  fir_dbl_col10/28(imag_back_out6) -> fir_dbl_col9/28(imag_back6)
  fir_dbl_col10/29(real_back_out7) -> fir_dbl_col9/29(real_back7)
  fir_dbl_col10/30(imag_back_out7) -> fir_dbl_col9/30(imag_back7)
  fir_dbl_col10/31(real_back_out8) -> fir_dbl_col9/31(real_back8)
  fir_dbl_col10/32(imag_back_out8) -> fir_dbl_col9/32(imag_back8)
  fir_dbl_col11/17(real_back_out1) -> fir_dbl_col10/17(real_back1)
  fir_dbl_col11/18(imag_back_out1) -> fir_dbl_col10/18(imag_back1)
  fir_dbl_col11/19(real_back_out2) -> fir_dbl_col10/19(real_back2)
  fir_dbl_col11/20(imag_back_out2) -> fir_dbl_col10/20(imag_back2)
  fir_dbl_col11/21(real_back_out3) -> fir_dbl_col10/21(real_back3)
  fir_dbl_col11/22(imag_back_out3) -> fir_dbl_col10/22(imag_back3)
  fir_dbl_col11/23(real_back_out4) -> fir_dbl_col10/23(real_back4)
  fir_dbl_col11/24(imag_back_out4) -> fir_dbl_col10/24(imag_back4)
  fir_dbl_col11/25(real_back_out5) -> fir_dbl_col10/25(real_back5)
  fir_dbl_col11/26(imag_back_out5) -> fir_dbl_col10/26(imag_back5)
  fir_dbl_col11/27(real_back_out6) -> fir_dbl_col10/27(real_back6)
  fir_dbl_col11/28(imag_back_out6) -> fir_dbl_col10/28(imag_back6)
  fir_dbl_col11/29(real_back_out7) -> fir_dbl_col10/29(real_back7)
  fir_dbl_col11/30(imag_back_out7) -> fir_dbl_col10/30(imag_back7)
  fir_dbl_col11/31(real_back_out8) -> fir_dbl_col10/31(real_back8)
  fir_dbl_col11/32(imag_back_out8) -> fir_dbl_col10/32(imag_back8)
  fir_dbl_col12/17(real_back_out1) -> fir_dbl_col11/17(real_back1)
  fir_dbl_col12/18(imag_back_out1) -> fir_dbl_col11/18(imag_back1)
  fir_dbl_col12/19(real_back_out2) -> fir_dbl_col11/19(real_back2)
  fir_dbl_col12/20(imag_back_out2) -> fir_dbl_col11/20(imag_back2)
  fir_dbl_col12/21(real_back_out3) -> fir_dbl_col11/21(real_back3)
  fir_dbl_col12/22(imag_back_out3) -> fir_dbl_col11/22(imag_back3)
  fir_dbl_col12/23(real_back_out4) -> fir_dbl_col11/23(real_back4)
  fir_dbl_col12/24(imag_back_out4) -> fir_dbl_col11/24(imag_back4)
  fir_dbl_col12/25(real_back_out5) -> fir_dbl_col11/25(real_back5)
  fir_dbl_col12/26(imag_back_out5) -> fir_dbl_col11/26(imag_back5)
  fir_dbl_col12/27(real_back_out6) -> fir_dbl_col11/27(real_back6)
  fir_dbl_col12/28(imag_back_out6) -> fir_dbl_col11/28(imag_back6)
  fir_dbl_col12/29(real_back_out7) -> fir_dbl_col11/29(real_back7)
  fir_dbl_col12/30(imag_back_out7) -> fir_dbl_col11/30(imag_back7)
  fir_dbl_col12/31(real_back_out8) -> fir_dbl_col11/31(real_back8)
  fir_dbl_col12/32(imag_back_out8) -> fir_dbl_col11/32(imag_back8)
  fir_dbl_col13/17(real_back_out1) -> fir_dbl_col12/17(real_back1)
  fir_dbl_col13/18(imag_back_out1) -> fir_dbl_col12/18(imag_back1)
  fir_dbl_col13/19(real_back_out2) -> fir_dbl_col12/19(real_back2)
  fir_dbl_col13/20(imag_back_out2) -> fir_dbl_col12/20(imag_back2)
  fir_dbl_col13/21(real_back_out3) -> fir_dbl_col12/21(real_back3)
  fir_dbl_col13/22(imag_back_out3) -> fir_dbl_col12/22(imag_back3)
  fir_dbl_col13/23(real_back_out4) -> fir_dbl_col12/23(real_back4)
  fir_dbl_col13/24(imag_back_out4) -> fir_dbl_col12/24(imag_back4)
  fir_dbl_col13/25(real_back_out5) -> fir_dbl_col12/25(real_back5)
  fir_dbl_col13/26(imag_back_out5) -> fir_dbl_col12/26(imag_back5)
  fir_dbl_col13/27(real_back_out6) -> fir_dbl_col12/27(real_back6)
  fir_dbl_col13/28(imag_back_out6) -> fir_dbl_col12/28(imag_back6)
  fir_dbl_col13/29(real_back_out7) -> fir_dbl_col12/29(real_back7)
  fir_dbl_col13/30(imag_back_out7) -> fir_dbl_col12/30(imag_back7)
  fir_dbl_col13/31(real_back_out8) -> fir_dbl_col12/31(real_back8)
  fir_dbl_col13/32(imag_back_out8) -> fir_dbl_col12/32(imag_back8)
  fir_dbl_col14/17(real_back_out1) -> fir_dbl_col13/17(real_back1)
  fir_dbl_col14/18(imag_back_out1) -> fir_dbl_col13/18(imag_back1)
  fir_dbl_col14/19(real_back_out2) -> fir_dbl_col13/19(real_back2)
  fir_dbl_col14/20(imag_back_out2) -> fir_dbl_col13/20(imag_back2)
  fir_dbl_col14/21(real_back_out3) -> fir_dbl_col13/21(real_back3)
  fir_dbl_col14/22(imag_back_out3) -> fir_dbl_col13/22(imag_back3)
  fir_dbl_col14/23(real_back_out4) -> fir_dbl_col13/23(real_back4)
  fir_dbl_col14/24(imag_back_out4) -> fir_dbl_col13/24(imag_back4)
  fir_dbl_col14/25(real_back_out5) -> fir_dbl_col13/25(real_back5)
  fir_dbl_col14/26(imag_back_out5) -> fir_dbl_col13/26(imag_back5)
  fir_dbl_col14/27(real_back_out6) -> fir_dbl_col13/27(real_back6)
  fir_dbl_col14/28(imag_back_out6) -> fir_dbl_col13/28(imag_back6)
  fir_dbl_col14/29(real_back_out7) -> fir_dbl_col13/29(real_back7)
  fir_dbl_col14/30(imag_back_out7) -> fir_dbl_col13/30(imag_back7)
  fir_dbl_col14/31(real_back_out8) -> fir_dbl_col13/31(real_back8)
  fir_dbl_col14/32(imag_back_out8) -> fir_dbl_col13/32(imag_back8)
  fir_dbl_col15/17(real_back_out1) -> fir_dbl_col14/17(real_back1)
  fir_dbl_col15/18(imag_back_out1) -> fir_dbl_col14/18(imag_back1)
  fir_dbl_col15/19(real_back_out2) -> fir_dbl_col14/19(real_back2)
  fir_dbl_col15/20(imag_back_out2) -> fir_dbl_col14/20(imag_back2)
  fir_dbl_col15/21(real_back_out3) -> fir_dbl_col14/21(real_back3)
  fir_dbl_col15/22(imag_back_out3) -> fir_dbl_col14/22(imag_back3)
  fir_dbl_col15/23(real_back_out4) -> fir_dbl_col14/23(real_back4)
  fir_dbl_col15/24(imag_back_out4) -> fir_dbl_col14/24(imag_back4)
  fir_dbl_col15/25(real_back_out5) -> fir_dbl_col14/25(real_back5)
  fir_dbl_col15/26(imag_back_out5) -> fir_dbl_col14/26(imag_back5)
  fir_dbl_col15/27(real_back_out6) -> fir_dbl_col14/27(real_back6)
  fir_dbl_col15/28(imag_back_out6) -> fir_dbl_col14/28(imag_back6)
  fir_dbl_col15/29(real_back_out7) -> fir_dbl_col14/29(real_back7)
  fir_dbl_col15/30(imag_back_out7) -> fir_dbl_col14/30(imag_back7)
  fir_dbl_col15/31(real_back_out8) -> fir_dbl_col14/31(real_back8)
  fir_dbl_col15/32(imag_back_out8) -> fir_dbl_col14/32(imag_back8)
  fir_dbl_col16/17(real_back_out1) -> fir_dbl_col15/17(real_back1)
  fir_dbl_col16/18(imag_back_out1) -> fir_dbl_col15/18(imag_back1)
  fir_dbl_col16/19(real_back_out2) -> fir_dbl_col15/19(real_back2)
  fir_dbl_col16/20(imag_back_out2) -> fir_dbl_col15/20(imag_back2)
  fir_dbl_col16/21(real_back_out3) -> fir_dbl_col15/21(real_back3)
  fir_dbl_col16/22(imag_back_out3) -> fir_dbl_col15/22(imag_back3)
  fir_dbl_col16/23(real_back_out4) -> fir_dbl_col15/23(real_back4)
  fir_dbl_col16/24(imag_back_out4) -> fir_dbl_col15/24(imag_back4)
  fir_dbl_col16/25(real_back_out5) -> fir_dbl_col15/25(real_back5)
  fir_dbl_col16/26(imag_back_out5) -> fir_dbl_col15/26(imag_back5)
  fir_dbl_col16/27(real_back_out6) -> fir_dbl_col15/27(real_back6)
  fir_dbl_col16/28(imag_back_out6) -> fir_dbl_col15/28(imag_back6)
  fir_dbl_col16/29(real_back_out7) -> fir_dbl_col15/29(real_back7)
  fir_dbl_col16/30(imag_back_out7) -> fir_dbl_col15/30(imag_back7)
  fir_dbl_col16/31(real_back_out8) -> fir_dbl_col15/31(real_back8)
  fir_dbl_col16/32(imag_back_out8) -> fir_dbl_col15/32(imag_back8)
  fir_dbl_col16/1(real_out1) -> fir_dbl_col16/17(real_back1)
  fir_dbl_col16/2(imag_out1) -> fir_dbl_col16/18(imag_back1)
  fir_dbl_col16/3(real_out2) -> fir_dbl_col16/19(real_back2)
  fir_dbl_col16/4(imag_out2) -> fir_dbl_col16/20(imag_back2)
  fir_dbl_col16/5(real_out3) -> fir_dbl_col16/21(real_back3)
  fir_dbl_col16/6(imag_out3) -> fir_dbl_col16/22(imag_back3)
  fir_dbl_col16/7(real_out4) -> fir_dbl_col16/23(real_back4)
  fir_dbl_col16/8(imag_out4) -> fir_dbl_col16/24(imag_back4)
  fir_dbl_col16/9(real_out5) -> fir_dbl_col16/25(real_back5)
  fir_dbl_col16/10(imag_out5) -> fir_dbl_col16/26(imag_back5)
  fir_dbl_col16/11(real_out6) -> fir_dbl_col16/27(real_back6)
  fir_dbl_col16/12(imag_out6) -> fir_dbl_col16/28(imag_back6)
  fir_dbl_col16/13(real_out7) -> fir_dbl_col16/29(real_back7)
  fir_dbl_col16/14(imag_out7) -> fir_dbl_col16/30(imag_back7)
  fir_dbl_col16/15(real_out8) -> fir_dbl_col16/31(real_back8)
  fir_dbl_col16/16(imag_out8) -> fir_dbl_col16/32(imag_back8)
